simulink model "ADC_reader_simulink"  (R2025a)
settings: Solver=FixedStepAuto  StartTime=0.0  StopTime=5  FixedStep=0.01  RelTol=1e-3  EnableMultiTasking=on
libraries: stm32f4xxblockslib x7, dspstat3 x1, eeGeneralControl x1
settings Model: STM32="{\"AnalogInput\":[{\"ID\":\"test_poten:20\"},{\"ID\":\"test_poten:28\"},{\"ID\":\"ADC_reader:28\"},{\"ID\":\"ADC_reader:20\"},{\"ID\":\"ADC_reader:14\"},{\"ID\":\"ADC_reader:11\"},{\"ID\":\"ADC_reader:8\"},{\"ID\":\"ADC_reader:5\"},{\"ID\":\"ADC_reader:1\"},{\"ID\":\"ADC_reader_simulink:14\"},{\"ID\":\"ADC_reader_simulink:11\"},{\"ID\":\"ADC_reader_simulink:8\"},{\"ID\":\"ADC_reader_simulink:5\"},{\"ID\":\"ADC_reader_simulink:1\"},{\"ID\":\"ADC_reader_simulink:20\"},{\"ID\":\"ADC_reader_simulink:28\"}]}"  Creator=ioonz  LastModifiedBy=fffif
settings OptimizationCC: DefaultParameterBehavior=Inlined  EnhancedBackFolding=on  PassReuseOutputArgsAs=Individual arguments  ZeroExternalMemoryAtStartup=off  ZeroInternalMemoryAtStartup=off  MaxStackSize=512  OptimizeBlockOrder=speed  DifferentSizesBufferReuse=on  OptimizationCustomize=off  EfficientTunableParamExpr=on
settings DebuggingCC: ParameterTunabilityLossMsg=error
settings HardwareCC: ProdBitPerPointer=32.0  ProdBitPerSizeT=32.0  ProdBitPerPtrDiffT=32.0  ProdLargestAtomicInteger=Long  ProdLargestAtomicFloat=Double  ProdWordSize=32.0  ProdLongLongMode=on  ProdHWDeviceType=ARM Compatible->ARM Cortex-M
settings SFSimCC: MATLABDynamicMemAlloc=off
settings RTWCC: SystemTargetFile=ert.tlc  HardwareBoard=STM32G4xx Based  TemplateMakefile=ert_default_tmf  Toolchain=GNU Tools for ARM Embedded Processors  Description=Embedded Coder
settings CodeAppCC: ForceParamTrailComments=on  IgnoreCustomStorageClasses=off  OperatorAnnotations=on  SimulinkDataObjDesc=on  SFDataObjDesc=on  InsertBlockDesc=on
settings ERTTargetCC: ExtModeTransport=3.0  ExtModeStaticAllocSize=2048.0  TargetLangStandard=C99 (ISO)  CodeReplacementLibrary=ARM Cortex-M

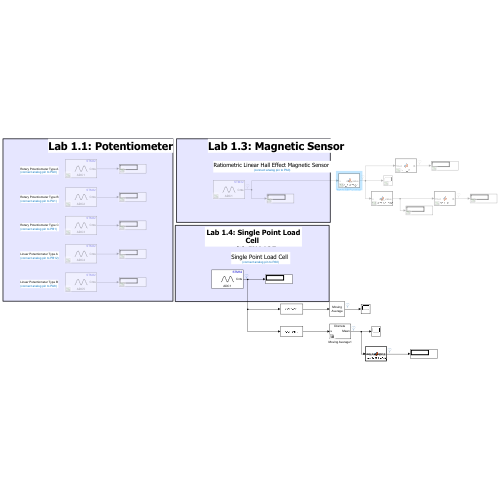
[thumbnail: Simulink's stored preview of the top-level diagram]
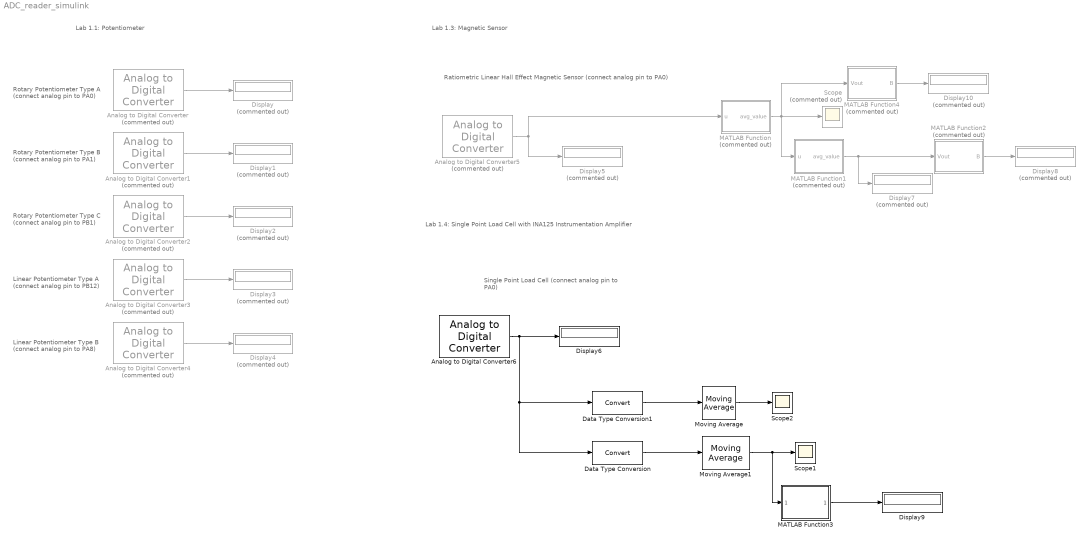
== system ADC_reader_simulink ==
  note: Lab 1.1: Potentiometer
  note: Rotary Potentiometer Type A
      | (connect analog pin to PA0)
  note: Rotary Potentiometer Type B
      | (connect analog pin to PA1)
  note: Rotary Potentiometer Type C
      | (connect analog pin to PB1)
  note: Linear Potentiometer Type A
      | (connect analog pin to PB12)
  note: Linear Potentiometer Type B
      | (connect analog pin to PA8)
  note: Ratiometric Linear Hall Effect Magnetic Sensor
      | (connect analog pin to PA0)
  note: Single Point Load Cell
      | (connect analog pin to PA0)
  note: Lab 1.3: Magnetic Sensor
  note: Lab 1.4: Single Point Load Cell
      | with INA125 Instrumentation Amplifier
  Analog to Digital Converter : stm32f4xxblockslib/Analog to Digital Converter  Commented=on  ADCModule=ADC1  ConversionGroup=Regular  TriggerMode=Trigger and read  NumberOfConversions=1  EnableBufferConv=off  BufferLength=1  OutputStatus=off  SampleTime=-1  EnableSimPort=off  hoistedMaskSrc=ECSoC/ECSimCodegen/Analog to Digital Converter
  Analog to Digital Converter1 : stm32f4xxblockslib/Analog to Digital Converter  Commented=on  ADCModule=ADC2  ConversionGroup=Regular  TriggerMode=Trigger and read  NumberOfConversions=1  EnableBufferConv=off  BufferLength=1  OutputStatus=off  SampleTime=-1  EnableSimPort=off  hoistedMaskSrc=ECSoC/ECSimCodegen/Analog to Digital Converter
  Analog to Digital Converter2 : stm32f4xxblockslib/Analog to Digital Converter  Commented=on  ADCModule=ADC3  ConversionGroup=Regular  TriggerMode=Trigger and read  NumberOfConversions=1  EnableBufferConv=off  BufferLength=1  OutputStatus=off  SampleTime=-1  EnableSimPort=off  hoistedMaskSrc=ECSoC/ECSimCodegen/Analog to Digital Converter
  Analog to Digital Converter3 : stm32f4xxblockslib/Analog to Digital Converter  Commented=on  ADCModule=ADC4  ConversionGroup=Regular  TriggerMode=Trigger and read  NumberOfConversions=1  EnableBufferConv=off  BufferLength=1  OutputStatus=off  SampleTime=-1  EnableSimPort=off  hoistedMaskSrc=ECSoC/ECSimCodegen/Analog to Digital Converter
  Analog to Digital Converter4 : stm32f4xxblockslib/Analog to Digital Converter  Commented=on  ADCModule=ADC5  ConversionGroup=Regular  TriggerMode=Trigger and read  NumberOfConversions=1  EnableBufferConv=off  BufferLength=1  OutputStatus=off  SampleTime=-1  EnableSimPort=off  hoistedMaskSrc=ECSoC/ECSimCodegen/Analog to Digital Converter
  Analog to Digital Converter5 : stm32f4xxblockslib/Analog to Digital Converter  Commented=on  ADCModule=ADC1  ConversionGroup=Regular  TriggerMode=Trigger and read  NumberOfConversions=1  EnableBufferConv=off  BufferLength=1  OutputStatus=off  SampleTime=-1  EnableSimPort=off  hoistedMaskSrc=ECSoC/ECSimCodegen/Analog to Digital Converter
  Analog to Digital Converter6 : stm32f4xxblockslib/Analog to Digital Converter  ADCModule=ADC1  ConversionGroup=Regular  TriggerMode=Trigger and read  NumberOfConversions=1  EnableBufferConv=off  BufferLength=1  OutputStatus=off  SampleTime=-1  EnableSimPort=off  hoistedMaskSrc=ECSoC/ECSimCodegen/Analog to Digital Converter
  Data Type Conversion : DataTypeConversion  SaturateOnIntegerOverflow=off  RndMeth=Floor
  Data Type Conversion1 : DataTypeConversion  SaturateOnIntegerOverflow=off  RndMeth=Floor
  Display{,1..5,7..8,10} (9 alike) : Display  Commented=on
  Display6 : Display
  Display9 : Display
  MATLAB Function : MATLAB Function  Commented=on  TreatAsAtomicUnit=on
  MATLAB Function1 : MATLAB Function  Commented=on  TreatAsAtomicUnit=on
  MATLAB Function2 : MATLAB Function  Commented=on  TreatAsAtomicUnit=on
  MATLAB Function3 : MATLAB Function  TreatAsAtomicUnit=on
  MATLAB Function4 : MATLAB Function  Commented=on  TreatAsAtomicUnit=on
  Moving Average : dspstat3/Moving Average  Method=Sliding window  ForgettingFactorPort=off  SpecifyWindowLength=on  WindowLength=4  OverlapLength=3  AllowArbitraryInputLength=off  ForgettingFactor=0.9  SimulateUsing=Interpreted execution
  Moving Average1 : eeGeneralControl/Moving Average  VariantControl=Variant1  LabelModeActiveChoice=Discrete  f=60  x0=0  BufferSize=8192  Ts=-1
      settings: LibrarySourceBlock=ee_sl_lib/General Control/Moving Average
  Scope : Scope  Commented=on
      settings: ActiveDisplayYMinimum=3233.2711054918664  ActiveDisplayYMaximum=3337.5789847997457
  Scope1 : Scope
      settings: ActiveDisplayYMinimum=-8.9749999999998362  ActiveDisplayYMaximum=80.774999999998542
  Scope2 : Scope
      settings: ActiveDisplayYMinimum=450.9092271818788  ActiveDisplayYMaximum=2471.8169553630914  DataLoggingVariableName=ScopeData2
  wires:
  Analog to Digital Converter/1 -> Display/1
  Analog to Digital Converter1/1 -> Display1/1
  Analog to Digital Converter2/1 -> Display2/1
  Analog to Digital Converter3/1 -> Display3/1
  Analog to Digital Converter4/1 -> Display4/1
  Analog to Digital Converter5/1 -> Display5/1, MATLAB Function/1(u)
  MATLAB Function/1(avg_value) -> MATLAB Function4/1(Vout), MATLAB Function1/1(u), Scope/1
  MATLAB Function1/1(avg_value) -> Display7/1, MATLAB Function2/1(Vout)
  MATLAB Function2/1(B) -> Display8/1
  Moving Average1/1 -> MATLAB Function3/1(avg_adc_signal), Scope1/1
  Data Type Conversion/1 -> Moving Average1/1
  Data Type Conversion1/1 -> Moving Average/1
  Analog to Digital Converter6/1 -> Data Type Conversion/1, Data Type Conversion1/1, Display6/1
  Moving Average/1 -> Scope2/1
  MATLAB Function3/1(calculated_weight_g) -> Display9/1
  MATLAB Function4/1(B) -> Display10/1

== matlab function ADC_reader_simulink/MATLAB Function ==
  data: u input; avg_value output
function avg_value = adc_average(u)

persistent sumVal count 

if isempty(sumVal)
    sumVal = 0;     
    count = 0;      
end

sumVal = sumVal + double(u);
count = count + 1;

avg_value = sumVal / count; 
end

== matlab function ADC_reader_simulink/MATLAB Function2 ==
  data: Vout input; B output
function B = find_B(Vout)
    % Constants
    VQ = 3.3/2;                      % ตัวอย่างค่า offset voltage (V)
    Sensitivity_25C = 1.3;         % Sensitivity ที่ 25°C (mV/G)
    STC = 0.001;                   % Sensitivity temperature coefficient (per °C)
    TA = 26;                       % Ambient temperature (°C)

    % Calculation
    B = (Vout - VQ) ./ (Sensitivity_25C * (1 + STC * (TA - 25)));
end

== matlab function ADC_reader_simulink/MATLAB Function3 ==
  data: avg_adc_signal input; calculated_weight_g output
function calculated_weight_g = convertADCtoWeight(avg_adc_signal)

% โดยใช้สมการ Calibration (y = mx + c)

m_slope  = 1906562422;3.08549
c_offset = -3.236277211858530e+02;

%    ผลลัพธ์ตรงนี้คือ "ค่าฝั่งขวา" ในตารางของคุณ
incorrect_weight_g = (m_slope * avg_adc_signal) + c_offset;

% อัตราส่วนของน้ำหนักที่ error เมื่อเทียบกับน้ำหนักที่ถูกต้อง
calculated_weight_g = (incorrect_weight_g + 200) / 1.2;

if calculated_weight_g < 0
    calculated_weight_g = 0;
end
end

== matlab function ADC_reader_simulink/MATLAB Function4 ==
  data: Vout input; B output
function B = find_B(Vout)
    % Constants
    VQ = 3.3/2;                      % ตัวอย่างค่า offset voltage (V)
    Sensitivity_25C = 1.3;         % Sensitivity ที่ 25°C (mV/G)
    STC = 0.001;                   % Sensitivity temperature coefficient (per °C)
    TA = 26;                       % Ambient temperature (°C)

    % Calculation
    B = (Vout - VQ) ./ (Sensitivity_25C * (1 + STC * (TA - 25)));
end

== matlab function ADC_reader_simulink/MATLAB Function1 ==
  data: u input; avg_value output
function avg_value = adc_average_single(u)
%  u - ADC reading (e.g., 0–4095)
%  avg_value - final average value 
Vref = 3.3;
ADC_max = 4095;
Nmax = 1000;   

persistent sumVal count avgVal done

if isempty(sumVal)
    sumVal = 0;     
    count  = 0;     
    avgVal = 0;     
    done   = false; 
end

if ~done
    % mV
    Vout_mV = (double(u) / ADC_max) * Vref * 1000;

    sumVal = sumVal + Vout_mV;
    count  = count + 1;

    % compute average
    if count >= Nmax
        avgVal = sumVal / count;
        done = true; 
    end
end

% Output
avg_value = avgVal;

end
